simulink model "solution1"  (R2017b)
settings: Solver=VariableStepAuto  StartTime=0.0  StopTime=25  FixedStep=0.1  MaxStep=1e-1  RelTol=1e-3  AbsTol=1e-3
libraries: simulink x7
settings Model: Creator=ashwin.ramanujam  LastModifiedBy=otkup

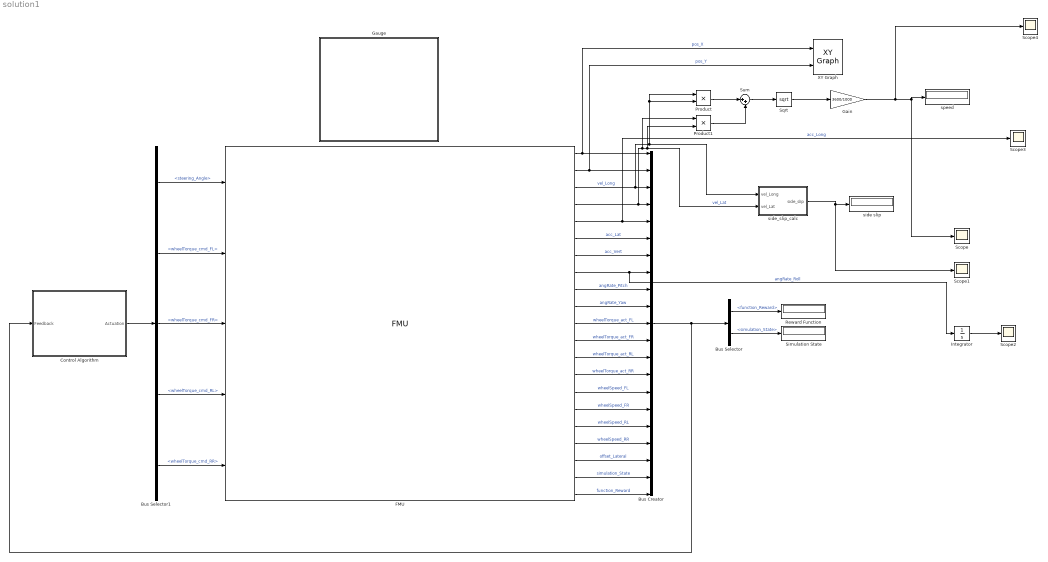
== system solution1 ==
  Bus Creator : BusCreator  Inputs=21
  Bus Selector : BusSelector  OutputSignals=function_Reward,simulation_State
  Bus Selector1 : BusSelector  OutputSignals=steering_Angle,wheelTorque_cmd_FL,wheelTorque_cmd_FR,wheelTorque_cmd_RL,wheelTorque_cmd_RR
  Control Algorithm : Subsystem
  FMU : FMU  FMUName=MED2018_VehicleModel.fmu  FMUDebugLogging=on  FMUMode=CoSimulation  FMUSampleTime=-1  mask(MED2018.VehicleModel [Co-Simulation, v2.0]){}
      mask Display:
      | if (exist([Simulink.fileGenControl('get','CacheFolder') '\slprj\_fmu\e4d23254ffb0d907ce810887e987e94d\MED2018_VehicleModel\model.png'],'file'))
      |     image([Simulink.fileGenControl('get','CacheFolder') '\slprj\_fmu\e4d23254ffb0d907ce810887e987e94d\MED2018_VehicleModel\model.png']);
      |     text(0.03, 0.97, 'MED2018.VehicleModel', 'horizontalAlignment', 'left', 'verticalAlignment', 'top');
      | else
      |     disp('MED2018.VehicleModel');
      | end
      | port_label('output',1,'pos_X');
      | port_label('output',2,'pos_Y');
      | port_label('output',3,'vel_Long');
      | port_label('output',4,'vel_Lat');
      | port_label('output',5,'acc_Long');
      | port_label('output',6,'acc_Lat');
      | port_label('output',7,'acc_Vert');
      | port_label('output',8,'angRate_Roll');
      | port_label('output',9,'angRate_Pitch');
      | port_label('output',10,'angRate_Yaw');
      | port_label('output',11,'wheellTorque_act_FL');
      | port_label('output',12,'wheelTorque_act_FR');
      | port_label('output',13,'wheelTorque_act_RL');
      | port_label('output',14,'wheelTorque_act_RR');
      | port_label('output',15,'wheelSpeed_FL');
      | port_label('output',16,'wheelSpeed_FR');
      | port_label('output',17,'wheelSpeed_RL');
      | port_label('output',18,'wheelSpeed_RR');
      | port_label('output',19,'offset_Lateral');
      | port_label('output',20,'simulation_State');
      | port_label('output',21,'function_Reward');
      | port_label('input',1,'steering_Angle');
      | port_label('input',2,'wheelTorque_cmd_FL');
      | port_label('input',3,'wheelTorque_cmd_FR');
      | port_label('input',4,'wheelTorque_cmd_RL');
      | port_label('input',5,'wheelTorque_cmd_RR');
  Gain : Gain  Gain=3600/1000
  Gauge : Subsystem  DialogController=hmiCreateDDGDialog  IsWebBlock=on  mask(MWDashboardBlock){webBlockId=95ecb222-2df1-432b-9766-14efc8d26a24, webBlockType=circulargauge, ShowInLibBrowser=on, ShowInitialText=on, HMISrcModelName=solution1}
      mask prompts: webBlockId "WebBlock Id"; webBlockType "WebBlock Type"; HMISrcModelName "Source Model"
      mask help: SimulinkHMI:dialogs:CircularGaugeDialogDesc
      mask Help: helpview([docroot '/mapfiles/simulink.map'], 'hmi_gauge')
      mask Display:
      | if strcmp(get_param(bdroot(gcb),'BlockDiagramType'), 'library')
      |     image([(matlabroot) '/toolbox/simulink/hmi/icons/CircularGauge.png']);
      | end
  Integrator : Integrator
  Product : Product
  Product1 : Product
  Reward Function : Display
  Scope{,1..4} (5 alike) : Scope
  Simulation State : Display
  Sqrt : Sqrt  SaturateOnIntegerOverflow=on
  Sum : Sum  Inputs=|++
  XY Graph : simulink/Sinks/XY Graph  xmin=-100  xmax=200  ymin=-100  ymax=200  st=-1
  "side slip " : Display
  side_slip_calc : Subsystem
  "speed " : Display
  wires:
  Control Algorithm/1(Actuation) -> Bus Selector1/1
  Bus Selector1/1 -> FMU/1  "<steering_Angle>"
  Bus Selector1/2 -> FMU/2  "<wheelTorque_cmd_FL>"
  Bus Selector1/3 -> FMU/3  "<wheelTorque_cmd_FR>"
  Bus Selector1/4 -> FMU/4  "<wheelTorque_cmd_RL>"
  Bus Selector1/5 -> FMU/5  "<wheelTorque_cmd_RR>"
  FMU/1 -> XY Graph/1, Bus Creator/1  "pos_X"
  FMU/2 -> XY Graph/2, Bus Creator/2  "pos_Y"
  FMU/3 -> side_slip_calc/1(vel_Long), Product/2, Product/1, Bus Creator/3  "vel_Long"
  FMU/4 -> Product1/1, side_slip_calc/2(vel_Lat), Product1/2, Bus Creator/4  "vel_Lat"
  FMU/5 -> Scope3/1, Bus Creator/5  "acc_Long"
  FMU/6 -> Bus Creator/6  "acc_Lat"
  FMU/7 -> Bus Creator/7  "acc_Vert"
  FMU/8 -> Integrator/1, Bus Creator/8  "angRate_Roll"
  FMU/9 -> Bus Creator/9  "angRate_Pitch"
  FMU/10 -> Bus Creator/10  "angRate_Yaw"
  FMU/11 -> Bus Creator/11  "wheelTorque_act_FL"
  FMU/12 -> Bus Creator/12  "wheelTorque_act_FR"
  FMU/13 -> Bus Creator/13  "wheelTorque_act_RL"
  FMU/14 -> Bus Creator/14  "wheelTorque_act_RR"
  FMU/15 -> Bus Creator/15  "wheelSpeed_FL"
  FMU/16 -> Bus Creator/16  "wheelSpeed_FR"
  FMU/17 -> Bus Creator/17  "wheelSpeed_RL"
  FMU/18 -> Bus Creator/18  "wheelSpeed_RR"
  FMU/19 -> Bus Creator/19  "offset_Lateral"
  FMU/20 -> Bus Creator/20  "simulation_State"
  FMU/21 -> Bus Creator/21  "function_Reward"
  Bus Creator/1 -> Bus Selector/1, Control Algorithm/1(Feedback)
  Bus Selector/1 -> Reward Function/1  "<function_Reward>"
  Bus Selector/2 -> Simulation State/1  "<simulation_State>"
  Product1/1 -> Sum/2
  Product/1 -> Sum/1
  Sum/1 -> Sqrt/1
  Sqrt/1 -> Gain/1
  Gain/1 -> Scope4/1, "speed "/1, Scope/1
  Integrator/1 -> Scope2/1
  side_slip_calc/1(side_slip) -> Scope1/1, "side slip "/1

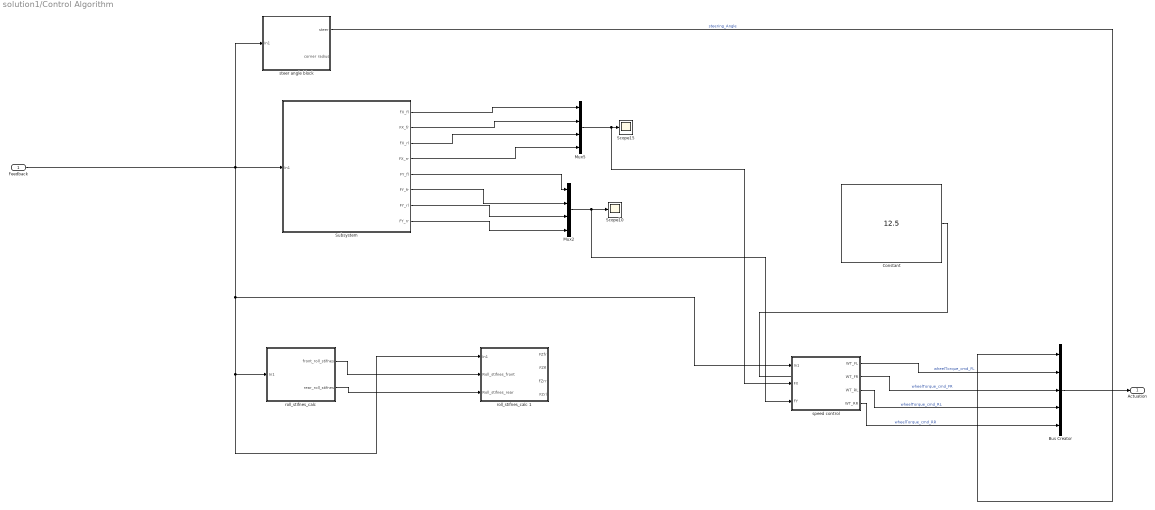
== system solution1/Control Algorithm ==
  Feedback : Inport
  Bus Creator : BusCreator  Inputs=5
  Constant : Constant  Value=12.5
  Mux2 : Mux
  Mux5 : Mux
  Scope10 : Scope
  Scope15 : Scope
  Subsystem : Subsystem
  "roll_stifnes_calc " : Subsystem
  roll_stifnes_calc 1 : Subsystem
  speed control : Subsystem
  "steer angle block " : Subsystem
  Actuation : Outport
  wires:
  speed control/4(WT_RR) -> Bus Creator/5  "wheelTorque_cmd_RR"
  speed control/1("WT_FL ") -> Bus Creator/2  "wheelTorque_cmd_FL"
  speed control/3(WT_RL) -> Bus Creator/4  "wheelTorque_cmd_RL"
  "steer angle block "/1("steer ") -> Bus Creator/1  "steering_Angle"
  speed control/2(WT_FR) -> Bus Creator/3  "wheelTorque_cmd_FR"
  Bus Creator/1 -> Actuation/1
  "roll_stifnes_calc "/1(front_roll_stifnes) -> roll_stifnes_calc 1/2(Roll_stifnes_front)
  "roll_stifnes_calc "/2(rear_roll_stifnes) -> roll_stifnes_calc 1/3("Roll_stifnes_rear ")
  Feedback/1 -> speed control/1(In1), roll_stifnes_calc 1/1(In1), "roll_stifnes_calc "/1(In1), "steer angle block "/1(In1), Subsystem/1(In1)
  Constant/1 -> ?
  Mux5/1 -> speed control/2(FX), Scope15/1
  Mux2/1 -> speed control/3(FY), Scope10/1
  Subsystem/1(FX_fl) -> Mux5/1
  Subsystem/2(FX_fr) -> Mux5/2
  Subsystem/3(FX_rl) -> Mux5/3
  Subsystem/4(FX_rr) -> Mux5/4
  Subsystem/5(FY_fl) -> Mux2/1
  Subsystem/6(FY_fr) -> Mux2/2
  Subsystem/7(FY_rl) -> Mux2/3
  Subsystem/8(FY_rr) -> Mux2/4

== system solution1/Gauge ==

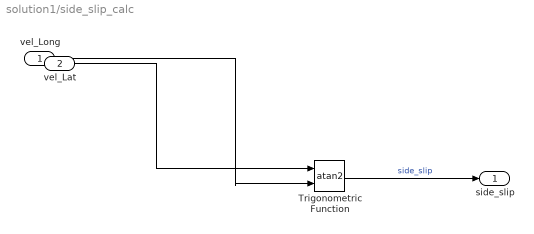
== system solution1/side_slip_calc ==
  vel_Long : Inport
  vel_Lat : Inport  Port=2
  Trigonometric Function : Trigonometry  Operator=atan2
  side_slip : Outport
  wires:
  Trigonometric Function/1 -> side_slip/1  "side_slip"
  vel_Lat/1 -> Trigonometric Function/1
  vel_Long/1 -> Trigonometric Function/2

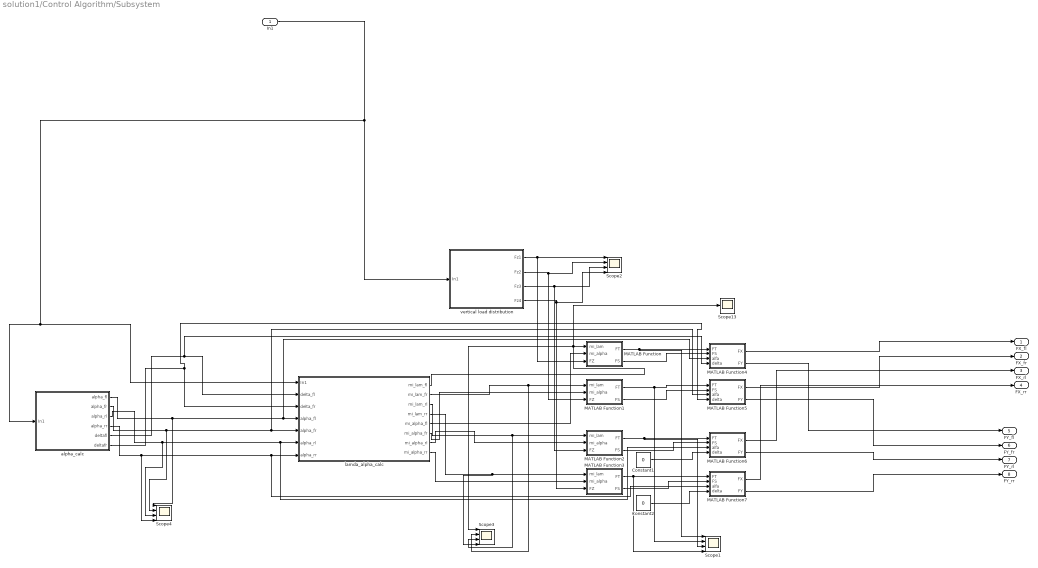
== system solution1/Control Algorithm/Subsystem ==
  In1 : Inport
  Constant1 : Constant  Value=0
  Constant2 : Constant  Value=0
  MATLAB Function : MATLAB Function  TreatAsAtomicUnit=on
  MATLAB Function1 : MATLAB Function  TreatAsAtomicUnit=on
  MATLAB Function2 : MATLAB Function  TreatAsAtomicUnit=on
  MATLAB Function3 : MATLAB Function  TreatAsAtomicUnit=on
  MATLAB Function4 : MATLAB Function  TreatAsAtomicUnit=on
  MATLAB Function5 : MATLAB Function  TreatAsAtomicUnit=on
  MATLAB Function6 : MATLAB Function  TreatAsAtomicUnit=on
  MATLAB Function7 : MATLAB Function  TreatAsAtomicUnit=on
  Scope{1..4} (4 alike) : Scope  NumInputPorts=4
  Scope13 : Scope
  alpha_calc : Subsystem
  lamda_alpha_calc : Subsystem
  vertical load distribution : Subsystem
  FX_fl : Outport
  FX_fr : Outport  Port=2
  FX_rl : Outport  Port=3
  FX_rr : Outport  Port=4
  FY_fl : Outport  Port=5
  FY_fr : Outport  Port=6
  FY_rl : Outport  Port=7
  FY_rr : Outport  Port=8
  wires:
  MATLAB Function/1(FT) -> Scope1/1, MATLAB Function4/1(FT)
  MATLAB Function6/2(FY) -> FY_rl/1
  MATLAB Function4/1(FX) -> FX_fl/1
  MATLAB Function6/1(FX) -> FX_rl/1
  MATLAB Function4/2(FY) -> FY_fl/1
  Constant1/1 -> MATLAB Function6/4(delta)
  vertical load distribution/3(Fz3) -> Scope2/3, MATLAB Function2/3(FZ)
  vertical load distribution/2(Fz2) -> Scope2/2, MATLAB Function1/3(FZ)
  alpha_calc/5(deltafl) -> MATLAB Function4/4(delta), lamda_alpha_calc/2(delta_fl)
  alpha_calc/6(deltafr) -> MATLAB Function5/4(delta), lamda_alpha_calc/3(delta_fr)
  vertical load distribution/4(Fz4) -> Scope2/4, MATLAB Function3/3(FZ)
  vertical load distribution/1(Fz1) -> Scope2/1, MATLAB Function/3(FZ)
  alpha_calc/3(alpha_rl) -> Scope4/3, MATLAB Function6/3(alfa), lamda_alpha_calc/6(alpha_rl)
  alpha_calc/2(alpha_fr) -> Scope4/2, MATLAB Function5/3(alfa), lamda_alpha_calc/5(alpha_fr)
  alpha_calc/4(alpha_rr) -> Scope4/4, MATLAB Function7/3(alfa), lamda_alpha_calc/7(alpha_rr)
  MATLAB Function3/1(FT) -> Scope1/4, MATLAB Function7/1(FT)
  MATLAB Function2/2(FS) -> MATLAB Function6/2(FS)
  MATLAB Function1/2(FS) -> MATLAB Function5/2(FS)
  MATLAB Function/2(FS) -> MATLAB Function4/2(FS)
  lamda_alpha_calc/4(mi_lam_rr) -> Scope3/4, MATLAB Function3/1(mi_lam)
  MATLAB Function5/1(FX) -> FX_fr/1
  MATLAB Function7/1(FX) -> FX_rr/1
  MATLAB Function5/2(FY) -> FY_fr/1
  lamda_alpha_calc/2(mi_lam_fr) -> Scope3/2, MATLAB Function1/1(mi_lam)
  lamda_alpha_calc/6(mi_alpha_fr) -> MATLAB Function1/2(mi_alpha)
  MATLAB Function7/2(FY) -> FY_rr/1
  MATLAB Function2/1(FT) -> Scope1/3, MATLAB Function6/1(FT)
  MATLAB Function1/1(FT) -> Scope1/2, MATLAB Function5/1(FT)
  lamda_alpha_calc/5(mi_alpha_fl) -> MATLAB Function/2(mi_alpha)
  In1/1 -> alpha_calc/1(In1), lamda_alpha_calc/1(In1), vertical load distribution/1(In1)
  lamda_alpha_calc/7(mi_alpha_rl) -> MATLAB Function2/2(mi_alpha)
  lamda_alpha_calc/3(mi_lam_rl) -> Scope3/3, MATLAB Function2/1(mi_lam)
  lamda_alpha_calc/8(mi_alpha_rr) -> MATLAB Function3/2(mi_alpha)
  MATLAB Function3/2(FS) -> MATLAB Function7/2(FS)
  Constant2/1 -> MATLAB Function7/4(delta)
  lamda_alpha_calc/1("mi_lam_fl ") -> Scope3/1, Scope13/1, MATLAB Function/1(mi_lam)
  alpha_calc/1(alpha_fl) -> Scope4/1, MATLAB Function4/3(alfa), lamda_alpha_calc/4(alpha_fl)

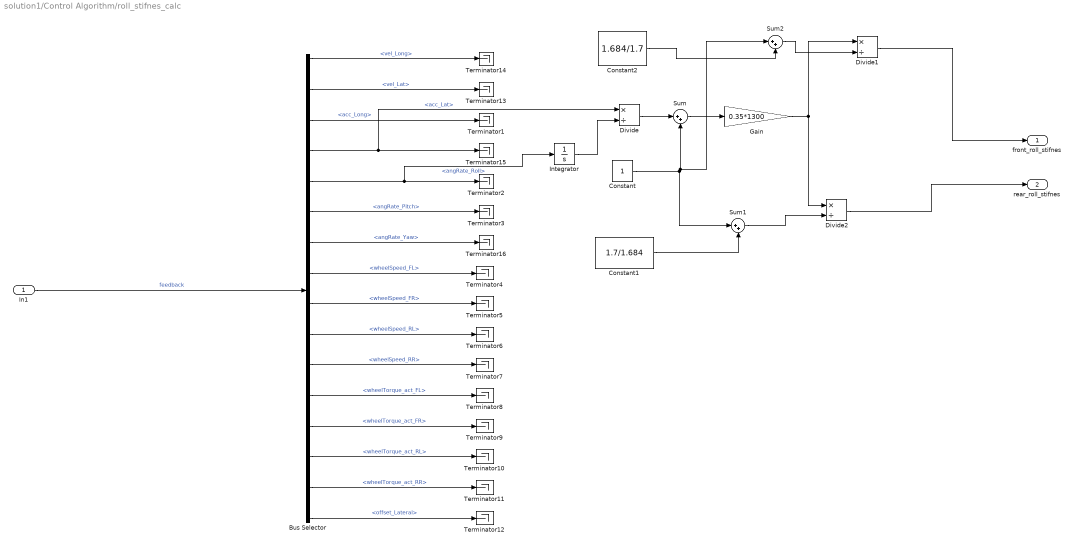
== system solution1/Control Algorithm/roll_stifnes_calc  ==
  In1 : Inport
  Bus Selector : BusSelector  OutputSignals=vel_Long,vel_Lat,acc_Long,acc_Lat,angRate_Roll,angRate_Pitch,angRate_Yaw,wheelSpeed_FL,wheelSpeed_FR,wheelSpeed_RL,wheelSpeed_RR,wheelTorque_act_FL,wheelTorque_act_FR,wheelTorque_act_RL,wheelTorque_act_RR,offset_Lateral
  Constant : Constant
  Constant1 : Constant  Value=1.7/1.684
  Constant2 : Constant  Value=1.684/1.7
  Divide : Product  Inputs=*/
  Divide1 : Product  Inputs=*/
  Divide2 : Product  Inputs=*/
  Gain : Gain  Gain=0.35*1300
  Integrator : Integrator
  Sum : Sum  Inputs=|++
  Sum1 : Sum  Inputs=|++
  Sum2 : Sum  Inputs=|++
  Terminator{1..16} (16 alike) : Terminator
  front_roll_stifnes : Outport
  rear_roll_stifnes : Outport  Port=2
  wires:
  Bus Selector/7 -> Terminator16/1  "<angRate_Yaw>"
  Bus Selector/4 -> Divide/1, Terminator15/1  "<acc_Lat>"
  Bus Selector/1 -> Terminator14/1  "<vel_Long>"
  In1/1 -> Bus Selector/1  "feedback"
  Bus Selector/13 -> Terminator9/1  "<wheelTorque_act_FR>"
  Bus Selector/5 -> Integrator/1, Terminator2/1  "<angRate_Roll>"
  Bus Selector/14 -> Terminator10/1  "<wheelTorque_act_RL>"
  Bus Selector/11 -> Terminator7/1  "<wheelSpeed_RR>"
  Bus Selector/12 -> Terminator8/1  "<wheelTorque_act_FL>"
  Bus Selector/16 -> Terminator12/1  "<offset_Lateral>"
  Bus Selector/15 -> Terminator11/1  "<wheelTorque_act_RR>"
  Bus Selector/9 -> Terminator5/1  "<wheelSpeed_FR>"
  Bus Selector/8 -> Terminator4/1  "<wheelSpeed_FL>"
  Bus Selector/10 -> Terminator6/1  "<wheelSpeed_RL>"
  Bus Selector/6 -> Terminator3/1  "<angRate_Pitch>"
  Bus Selector/3 -> Terminator1/1  "<acc_Long>"
  Bus Selector/2 -> Terminator13/1  "<vel_Lat>"
  Integrator/1 -> Divide/2
  Constant/1 -> Sum1/1, Sum2/1, Sum/2
  Divide/1 -> Sum/1
  Sum/1 -> Gain/1
  Gain/1 -> Divide2/1, Divide1/1
  Sum2/1 -> Divide1/2
  Sum1/1 -> Divide2/2
  Constant1/1 -> Sum1/2
  Constant2/1 -> Sum2/2
  Divide1/1 -> front_roll_stifnes/1
  Divide2/1 -> rear_roll_stifnes/1

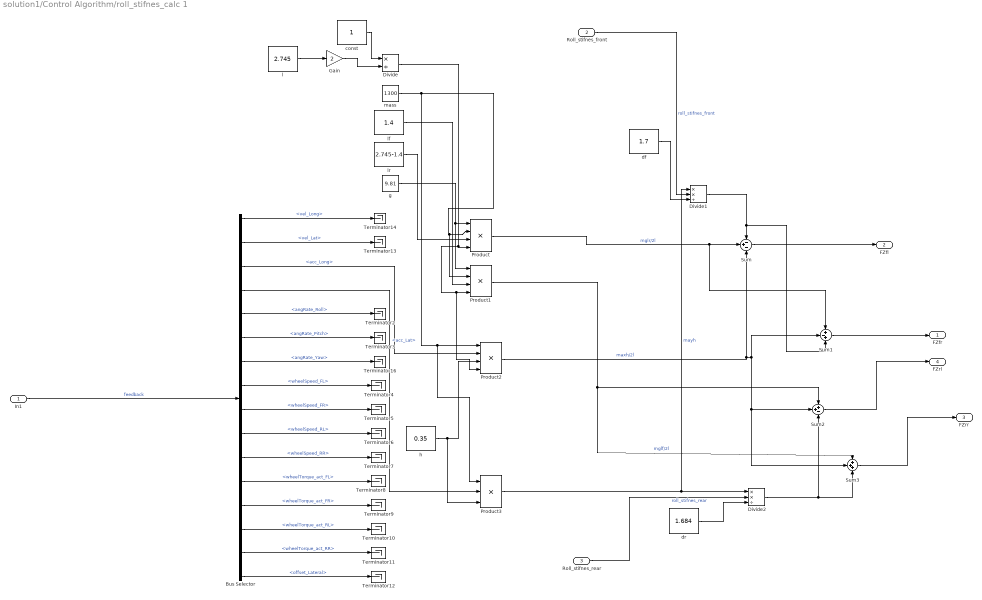
== system solution1/Control Algorithm/roll_stifnes_calc 1 ==
  In1 : Inport
  Roll_stifnes_front : Inport  Port=2
  "Roll_stifnes_rear " : Inport  Port=3
  Bus Selector : BusSelector  OutputSignals=vel_Long,vel_Lat,acc_Long,acc_Lat,angRate_Roll,angRate_Pitch,angRate_Yaw,wheelSpeed_FL,wheelSpeed_FR,wheelSpeed_RL,wheelSpeed_RR,wheelTorque_act_FL,wheelTorque_act_FR,wheelTorque_act_RL,wheelTorque_act_RR,offset_Lateral
  Divide : Product  Inputs=*/
  Divide1 : Product  Inputs=**/
  Divide2 : Product  Inputs=**/
  Gain : Gain  Gain=2
  Product : Product  Inputs=4
  Product1 : Product  Inputs=4
  Product2 : Product  Inputs=4
  Product3 : Product  Inputs=3
  Sum : Sum  Inputs=-+-
  Sum1 : Sum  Inputs=+-+
  Sum2 : Sum  Inputs=++-
  Sum3 : Sum  Inputs=+++
  Terminator{2..14,16} (14 alike) : Terminator
  const : Constant
  df : Constant  Value=1.7
  dr : Constant  Value=1.684
  g : Constant  Value=9.81
  h : Constant  Value=0.35
  "l " : Constant  Value=2.745
  "lf " : Constant  Value=1.4
  lr : Constant  Value=2.745-1.4
  mass : Constant  Value=1300
  FZfr : Outport
  FZfl : Outport  Port=2
  FZrr : Outport  Port=3
  FZrl : Outport  Port=4
  wires:
  Bus Selector/2 -> Terminator13/1  "<vel_Lat>"
  Bus Selector/3 -> Product2/2  "<acc_Long>"
  Bus Selector/6 -> Terminator3/1  "<angRate_Pitch>"
  Bus Selector/10 -> Terminator6/1  "<wheelSpeed_RL>"
  Bus Selector/8 -> Terminator4/1  "<wheelSpeed_FL>"
  Bus Selector/9 -> Terminator5/1  "<wheelSpeed_FR>"
  Bus Selector/15 -> Terminator11/1  "<wheelTorque_act_RR>"
  Bus Selector/16 -> Terminator12/1  "<offset_Lateral>"
  Bus Selector/12 -> Terminator8/1  "<wheelTorque_act_FL>"
  Bus Selector/11 -> Terminator7/1  "<wheelSpeed_RR>"
  Bus Selector/14 -> Terminator10/1  "<wheelTorque_act_RL>"
  Bus Selector/5 -> Terminator2/1  "<angRate_Roll>"
  Bus Selector/13 -> Terminator9/1  "<wheelTorque_act_FR>"
  In1/1 -> Bus Selector/1  "feedback"
  Bus Selector/1 -> Terminator14/1  "<vel_Long>"
  Bus Selector/4 -> Product3/2  "<acc_Lat>"
  Bus Selector/7 -> Terminator16/1  "<angRate_Yaw>"
  Roll_stifnes_front/1 -> Divide1/2  "roll_stifnes_front"
  "Roll_stifnes_rear "/1 -> Divide2/2  "roll_stifnes_rear"
  g/1 -> Product1/1, Product/1
  mass/1 -> Product3/1, Product2/1, Product1/2, Product/2
  lr/1 -> Product/3
  "lf "/1 -> Product1/3
  Product1/1 -> Sum3/1, Sum2/1  "mglf/2l"
  "l "/1 -> Gain/1
  const/1 -> Divide/1
  Gain/1 -> Divide/2
  Divide/1 -> Product2/4, Product1/4, Product/4
  h/1 -> Product3/3, Product2/3
  Product2/1 -> Sum3/2, Sum2/2, Sum1/2, Sum/3  "maxh/2l"
  Product3/1 -> Divide2/1, Divide1/1  "mayh"
  Sum/1 -> FZfl/1
  Product/1 -> Sum1/1, Sum/2  "mglr/2l"
  df/1 -> Divide1/3
  Divide1/1 -> Sum1/3, Sum/1
  Sum1/1 -> FZfr/1
  Sum2/1 -> FZrl/1
  Divide2/1 -> Sum3/3, Sum2/3
  dr/1 -> Divide2/3
  Sum3/1 -> FZrr/1

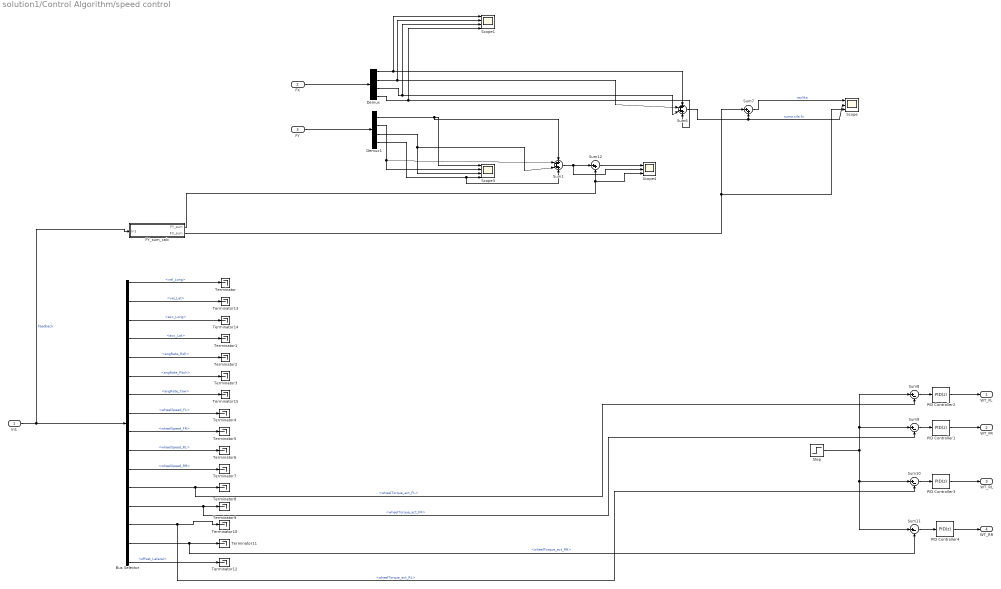
== system solution1/Control Algorithm/speed control ==
  In1 : Inport
  FX : Inport  Port=2
  FY : Inport  Port=3
  Bus Selector : BusSelector  OutputSignals=vel_Long,vel_Lat,acc_Long,acc_Lat,angRate_Roll,angRate_Pitch,angRate_Yaw,wheelSpeed_FL,wheelSpeed_FR,wheelSpeed_RL,wheelSpeed_RR,wheelTorque_act_FL,wheelTorque_act_FR,wheelTorque_act_RL,wheelTorque_act_RR,offset_Lateral
  Demux : Demux
  Demux1 : Demux
  FY_sum_calc : Subsystem
  PID Controller{1..4} (4 alike) : simulink/Continuous/PID Controller  Controller=PID  TimeDomain=Discrete-time  SampleTime=-1  IntegratorMethod=Forward Euler  FilterMethod=Forward Euler  Form=Parallel  UseFilter=on  ControllerParametersSource=internal  P=1  I=1.5  D=0  N=100  InitialConditionSource=internal  InitialConditionForIntegrator=0  InitialConditionForFilter=0  ExternalReset=none  LimitOutput=off  UpperSaturationLimit=inf  LowerSaturationLimit=-inf  LinearizeAsGain=on  AntiWindupMode=none  Kb=1  TrackingMode=off  Kt=1  PParamMin=[]  PParamMax=[]  IParamMin=[]  IParamMax=[]  DParamMin=[]  DParamMax=[]  NParamMin=[]  NParamMax=[]  KbParamMin=[]  KbParamMax=[]  KtParamMin=[]  KtParamMax=[]  POutMin=[]  POutMax=[]  IOutMin=[]  IOutMax=[]  DOutMin=[]  DOutMax=[]  NOutMin=[]  NOutMax=[]  KbOutMin=[]  KbOutMax=[]  KtOutMin=[]  KtOutMax=[]  IntegratorOutMin=[]  IntegratorOutMax=[]  FilterOutMin=[]  FilterOutMax=[]  SumOutMin=[]  SumOutMax=[]  SumI1OutMin=[]  SumI1OutMax=[]  SumI2OutMin=[]  SumI2OutMax=[]  SumI3OutMin=[]  SumI3OutMax=[]  SumDOutMin=[]  SumDOutMax=[]  SaturationOutMin=[]  SaturationOutMax=[]  IntegratorContinuousStateAttributes=''  IntegratorStateMustResolveToSignalObject=off  IntegratorRTWStateStorageClass=Auto  FilterContinuousStateAttributes=''  FilterStateMustResolveToSignalObject=off  FilterRTWStateStorageClass=Auto  DifferentiatorICPrevScaledInput=0  DifferentiatorOutMin=[]  DifferentiatorOutMax=[]  InitialConditionSetting=State (most efficient)  FilterDiffOutCoefMin=[]  FilterDiffOutCoefMax=[]  SumDenOutMin=[]  SumDenOutMax=[]  SumNumOutMin=[]  SumNumOutMax=[]  ReciprocalOutMin=[]  ReciprocalOutMax=[]  DivideOutMin=[]  DivideOutMax=[]  TunerSelectOption=Transfer Function Based (PID Tuner App)
  Scope : Scope  NumInputPorts=3
  Scope1 : Scope  NumInputPorts=4
  Scope3 : Scope  NumInputPorts=4
  Scope4 : Scope  NumInputPorts=3
  Step : Step  Time=15  Before=12.5  After=1000  SampleTime=0
  Sum1 : Sum  Inputs=++++
  Sum{8..11} (4 alike) : Sum  Inputs=|+-
  Sum12 : Sum  Inputs=|++
  Sum6 : Sum  Inputs=++++
  Sum7 : Sum  Inputs=|++
  Terminator{,1..15} (16 alike) : Terminator
  "WT_FL " : Outport
  WT_FR : Outport  Port=2
  WT_RL : Outport  Port=3
  WT_RR : Outport  Port=4
  wires:
  Bus Selector/7 -> Terminator15/1  "<angRate_Yaw>"
  Bus Selector/2 -> Terminator13/1  "<vel_Lat>"
  Bus Selector/3 -> Terminator14/1  "<acc_Long>"
  Bus Selector/6 -> Terminator3/1  "<angRate_Pitch>"
  Bus Selector/10 -> Terminator6/1  "<wheelSpeed_RL>"
  Bus Selector/8 -> Terminator4/1  "<wheelSpeed_FL>"
  Bus Selector/9 -> Terminator5/1  "<wheelSpeed_FR>"
  Bus Selector/15 -> Sum11/2, Terminator11/1  "<wheelTorque_act_RR>"
  Bus Selector/16 -> Terminator12/1  "<offset_Lateral>"
  Bus Selector/12 -> Sum8/2, Terminator8/1  "<wheelTorque_act_FL>"
  Bus Selector/11 -> Terminator7/1  "<wheelSpeed_RR>"
  Bus Selector/14 -> Sum10/2, Terminator10/1  "<wheelTorque_act_RL>"
  Bus Selector/1 -> Terminator/1  "<vel_Long>"
  Bus Selector/5 -> Terminator2/1  "<angRate_Roll>"
  Bus Selector/13 -> Sum9/2, Terminator9/1  "<wheelTorque_act_FR>"
  Bus Selector/4 -> Terminator1/1  "<acc_Lat>"
  In1/1 -> FY_sum_calc/1(In1), Bus Selector/1  "feedback"
  FX/1 -> Demux/1
  FY/1 -> Demux1/1
  Demux/1 -> Scope1/1, Sum6/1
  Demux/2 -> Scope1/2, Sum6/2
  Demux/3 -> Scope1/3, Sum6/3
  Sum7/1 -> Scope/1  "razlika"
  Sum6/1 -> Scope/2, Sum7/2  "suma sila fx"
  Sum10/1 -> PID Controller3/1
  Sum11/1 -> PID Controller4/1
  Sum9/1 -> PID Controller1/1
  Sum8/1 -> PID Controller2/1
  Step/1 -> Sum10/1, Sum11/1, Sum9/1, Sum8/1
  PID Controller2/1 -> "WT_FL "/1
  PID Controller1/1 -> WT_FR/1
  PID Controller3/1 -> WT_RL/1
  PID Controller4/1 -> WT_RR/1
  Demux/4 -> Scope1/4, Sum6/4
  Demux1/1 -> Sum1/1, Scope3/1
  Demux1/2 -> Sum1/2, Scope3/2
  Demux1/3 -> Sum1/3, Scope3/3
  Demux1/4 -> Sum1/4, Scope3/4
  Sum1/1 -> Scope4/2, Sum12/1
  FY_sum_calc/1(FY_sum) -> Scope4/3, Sum12/2
  Sum12/1 -> Scope4/1
  FY_sum_calc/2(FX_sum) -> Scope/3, Sum7/1

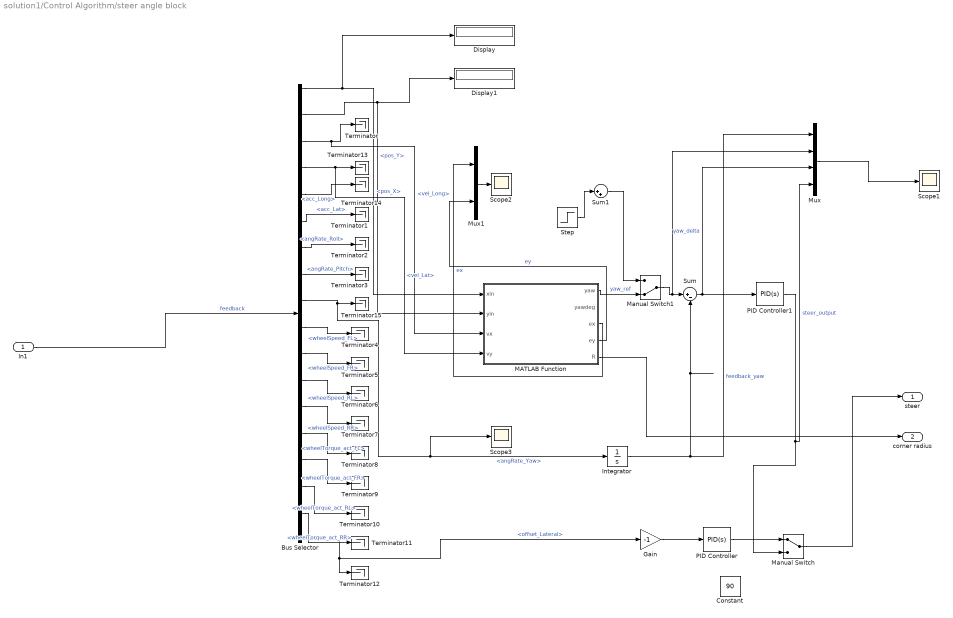
== system solution1/Control Algorithm/steer angle block  ==
  In1 : Inport
  Bus Selector : BusSelector  OutputSignals=pos_X,pos_Y,vel_Long,vel_Lat,acc_Long,acc_Lat,angRate_Roll,angRate_Pitch,angRate_Yaw,wheelSpeed_FL,wheelSpeed_FR,wheelSpeed_RL,wheelSpeed_RR,wheelTorque_act_FL,wheelTorque_act_FR,wheelTorque_act_RL,wheelTorque_act_RR,offset_Lateral
  Constant : Constant  Value=90
  Display : Display
  Display1 : Display
  Gain : Gain  Gain=-1
  Integrator : Integrator
  MATLAB Function : MATLAB Function  TreatAsAtomicUnit=on
  Manual Switch : ManualSwitch
  Manual Switch1 : ManualSwitch  CurrentSetting=0
  Mux : Mux
  Mux1 : Mux  Inputs=2
  PID Controller : simulink/Continuous/PID Controller  Controller=PID  TimeDomain=Continuous-time  SampleTime=-1  IntegratorMethod=Forward Euler  FilterMethod=Forward Euler  Form=Parallel  UseFilter=on  ControllerParametersSource=internal  P=1  I=0  D=1  N=100  InitialConditionSource=internal  InitialConditionForIntegrator=0  InitialConditionForFilter=0  ExternalReset=none  LimitOutput=off  UpperSaturationLimit=inf  LowerSaturationLimit=-inf  LinearizeAsGain=on  AntiWindupMode=none  Kb=1  TrackingMode=off  Kt=1  PParamMin=[]  PParamMax=[]  IParamMin=[]  IParamMax=[]  DParamMin=[]  DParamMax=[]  NParamMin=[]  NParamMax=[]  KbParamMin=[]  KbParamMax=[]  KtParamMin=[]  KtParamMax=[]  POutMin=[]  POutMax=[]  IOutMin=[]  IOutMax=[]  DOutMin=[]  DOutMax=[]  NOutMin=[]  NOutMax=[]  KbOutMin=[]  KbOutMax=[]  KtOutMin=[]  KtOutMax=[]  IntegratorOutMin=[]  IntegratorOutMax=[]  FilterOutMin=[]  FilterOutMax=[]  SumOutMin=[]  SumOutMax=[]  SumI1OutMin=[]  SumI1OutMax=[]  SumI2OutMin=[]  SumI2OutMax=[]  SumI3OutMin=[]  SumI3OutMax=[]  SumDOutMin=[]  SumDOutMax=[]  SaturationOutMin=[]  SaturationOutMax=[]  IntegratorContinuousStateAttributes=''  IntegratorStateMustResolveToSignalObject=off  IntegratorRTWStateStorageClass=Auto  FilterContinuousStateAttributes=''  FilterStateMustResolveToSignalObject=off  FilterRTWStateStorageClass=Auto  DifferentiatorICPrevScaledInput=0  DifferentiatorOutMin=[]  DifferentiatorOutMax=[]  InitialConditionSetting=State (most efficient)  FilterDiffOutCoefMin=[]  FilterDiffOutCoefMax=[]  SumDenOutMin=[]  SumDenOutMax=[]  SumNumOutMin=[]  SumNumOutMax=[]  ReciprocalOutMin=[]  ReciprocalOutMax=[]  DivideOutMin=[]  DivideOutMax=[]  TunerSelectOption=Transfer Function Based (PID Tuner App)
  PID Controller1 : simulink/Continuous/PID Controller  Controller=PID  TimeDomain=Continuous-time  SampleTime=-1  IntegratorMethod=Forward Euler  FilterMethod=Forward Euler  Form=Parallel  UseFilter=on  ControllerParametersSource=internal  P=12  I=0  D=0.2  N=0  InitialConditionSource=internal  InitialConditionForIntegrator=0  InitialConditionForFilter=0  ExternalReset=none  LimitOutput=off  UpperSaturationLimit=inf  LowerSaturationLimit=-inf  LinearizeAsGain=on  AntiWindupMode=none  Kb=1  TrackingMode=off  Kt=1  PParamMin=[]  PParamMax=[]  IParamMin=[]  IParamMax=[]  DParamMin=[]  DParamMax=[]  NParamMin=[]  NParamMax=[]  KbParamMin=[]  KbParamMax=[]  KtParamMin=[]  KtParamMax=[]  POutMin=[]  POutMax=[]  IOutMin=[]  IOutMax=[]  DOutMin=[]  DOutMax=[]  NOutMin=[]  NOutMax=[]  KbOutMin=[]  KbOutMax=[]  KtOutMin=[]  KtOutMax=[]  IntegratorOutMin=[]  IntegratorOutMax=[]  FilterOutMin=[]  FilterOutMax=[]  SumOutMin=[]  SumOutMax=[]  SumI1OutMin=[]  SumI1OutMax=[]  SumI2OutMin=[]  SumI2OutMax=[]  SumI3OutMin=[]  SumI3OutMax=[]  SumDOutMin=[]  SumDOutMax=[]  SaturationOutMin=[]  SaturationOutMax=[]  IntegratorContinuousStateAttributes=''  IntegratorStateMustResolveToSignalObject=off  IntegratorRTWStateStorageClass=Auto  FilterContinuousStateAttributes=''  FilterStateMustResolveToSignalObject=off  FilterRTWStateStorageClass=Auto  DifferentiatorICPrevScaledInput=0  DifferentiatorOutMin=[]  DifferentiatorOutMax=[]  InitialConditionSetting=State (most efficient)  FilterDiffOutCoefMin=[]  FilterDiffOutCoefMax=[]  SumDenOutMin=[]  SumDenOutMax=[]  SumNumOutMin=[]  SumNumOutMax=[]  ReciprocalOutMin=[]  ReciprocalOutMax=[]  DivideOutMin=[]  DivideOutMax=[]  TunerSelectOption=Transfer Function Based (PID Tuner App)
  Scope1 : Scope
  Scope2 : Scope
  Scope3 : Scope
  Step : Step  Time=0  After=0  SampleTime=0
  Sum : Sum  Inputs=|+-
  Sum1 : Sum  Inputs=|++
  Terminator{,1..15} (16 alike) : Terminator
  "steer " : Outport
  corner radius : Outport  Port=2
  wires:
  In1/1 -> Bus Selector/1  "feedback"
  Bus Selector/6 -> Terminator1/1  "<acc_Lat>"
  Bus Selector/15 -> Terminator9/1  "<wheelTorque_act_FR>"
  Bus Selector/7 -> Terminator2/1  "<angRate_Roll>"
  Bus Selector/3 -> MATLAB Function/3(vx), Terminator/1  "<vel_Long>"
  Bus Selector/16 -> Terminator10/1  "<wheelTorque_act_RL>"
  Bus Selector/13 -> Terminator7/1  "<wheelSpeed_RR>"
  Bus Selector/14 -> Terminator8/1  "<wheelTorque_act_FL>"
  Bus Selector/18 -> Terminator12/1, Gain/1  "<offset_Lateral>"
  Bus Selector/17 -> Terminator11/1  "<wheelTorque_act_RR>"
  Bus Selector/11 -> Terminator5/1  "<wheelSpeed_FR>"
  Bus Selector/10 -> Terminator4/1  "<wheelSpeed_FL>"
  Bus Selector/12 -> Terminator6/1  "<wheelSpeed_RL>"
  Bus Selector/8 -> Terminator3/1  "<angRate_Pitch>"
  Bus Selector/5 -> Terminator14/1  "<acc_Long>"
  Bus Selector/9 -> Scope3/1, Integrator/1, Terminator15/1  "<angRate_Yaw>"
  Gain/1 -> PID Controller/1
  PID Controller/1 -> Manual Switch/1
  Manual Switch/1 -> "steer "/1
  Integrator/1 -> Mux/1, Sum/2  "feedback_yaw"
  Sum/1 -> PID Controller1/1, Mux/3  "yaw_delta"
  Bus Selector/1 -> Display/1, MATLAB Function/1(xin)  "<pos_X>"
  Bus Selector/2 -> MATLAB Function/2(yin), Display1/1  "<pos_Y>"
  Bus Selector/4 -> MATLAB Function/4(vy), Terminator13/1  "<vel_Lat>"
  PID Controller1/1 -> Mux/4, Manual Switch/2  "steer_output"
  Mux/1 -> Scope1/1
  MATLAB Function/3(ex) -> Mux1/1  "ex"
  MATLAB Function/4(ey) -> Mux1/2  "ey"
  Mux1/1 -> Scope2/1
  MATLAB Function/1(yaw) -> Manual Switch1/2  "yaw_ref"
  Manual Switch1/1 -> Mux/2, Sum/1
  Step/1 -> Sum1/1
  Sum1/1 -> Manual Switch1/1
  MATLAB Function/5(R) -> corner radius/1

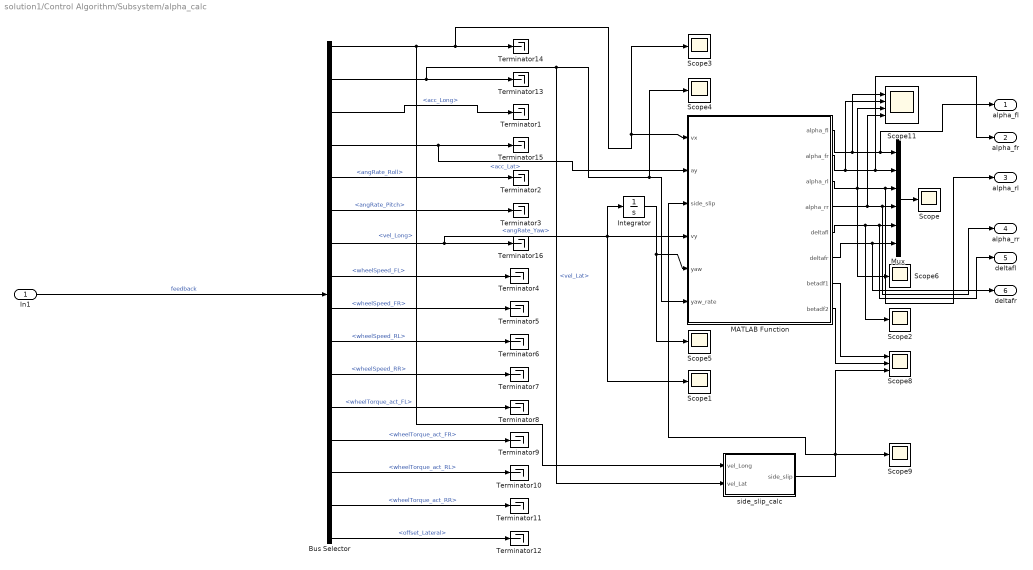
== system solution1/Control Algorithm/Subsystem/alpha_calc ==
  In1 : Inport
  Bus Selector : BusSelector  OutputSignals=vel_Long,vel_Lat,acc_Long,acc_Lat,angRate_Roll,angRate_Pitch,angRate_Yaw,wheelSpeed_FL,wheelSpeed_FR,wheelSpeed_RL,wheelSpeed_RR,wheelTorque_act_FL,wheelTorque_act_FR,wheelTorque_act_RL,wheelTorque_act_RR,offset_Lateral
  Integrator : Integrator
  MATLAB Function : MATLAB Function  TreatAsAtomicUnit=on
  Mux : Mux  Inputs=6
  Scope{,1..6,9} (8 alike) : Scope
  Scope11 : Scope  NumInputPorts=4
  Scope8 : Scope  NumInputPorts=3
  Terminator{1..16} (16 alike) : Terminator
  side_slip_calc : Subsystem
  alpha_fl : Outport
  alpha_fr : Outport  Port=2
  alpha_rl : Outport  Port=3
  alpha_rr : Outport  Port=4
  deltafl : Outport  Port=5
  deltafr : Outport  Port=6
  wires:
  Bus Selector/7 -> Scope1/1, Integrator/1, MATLAB Function/6(yaw_rate), Terminator16/1  "<angRate_Yaw>"
  Bus Selector/4 -> MATLAB Function/2(ay), Terminator15/1  "<acc_Lat>"
  Bus Selector/1 -> side_slip_calc/1(vel_Long), Scope3/1, MATLAB Function/1(vx), Terminator14/1  "<vel_Long>"
  In1/1 -> Bus Selector/1  "feedback"
  Bus Selector/13 -> Terminator9/1  "<wheelTorque_act_FR>"
  Bus Selector/5 -> Terminator2/1  "<angRate_Roll>"
  Bus Selector/14 -> Terminator10/1  "<wheelTorque_act_RL>"
  Bus Selector/11 -> Terminator7/1  "<wheelSpeed_RR>"
  Bus Selector/12 -> Terminator8/1  "<wheelTorque_act_FL>"
  Bus Selector/16 -> Terminator12/1  "<offset_Lateral>"
  Bus Selector/15 -> Terminator11/1  "<wheelTorque_act_RR>"
  Bus Selector/9 -> Terminator5/1  "<wheelSpeed_FR>"
  Bus Selector/8 -> Terminator4/1  "<wheelSpeed_FL>"
  Bus Selector/10 -> Terminator6/1  "<wheelSpeed_RL>"
  Bus Selector/6 -> Terminator3/1  "<angRate_Pitch>"
  Bus Selector/3 -> Terminator1/1  "<acc_Long>"
  Bus Selector/2 -> side_slip_calc/2(vel_Lat), Scope4/1, MATLAB Function/4(vy), Terminator13/1  "<vel_Lat>"
  Integrator/1 -> Scope5/1, MATLAB Function/5(yaw)
  MATLAB Function/1(alpha_fl) -> alpha_fl/1, Mux/1, Scope11/1
  MATLAB Function/2(alpha_fr) -> Scope11/2, alpha_fr/1, Mux/2
  MATLAB Function/3(alpha_rl) -> Scope11/3, alpha_rl/1, Mux/3, Scope6/1
  MATLAB Function/4(alpha_rr) -> alpha_rr/1, Mux/4, Scope11/4
  MATLAB Function/5(deltafl) -> Scope2/1, deltafl/1, Mux/5
  Mux/1 -> Scope/1
  side_slip_calc/1(side_slip) -> Scope8/3, Scope9/1, MATLAB Function/3(side_slip)
  MATLAB Function/7(betadf1) -> Scope8/1
  MATLAB Function/8(betadf2) -> Scope8/2
  MATLAB Function/6(deltafr) -> deltafr/1, Mux/6

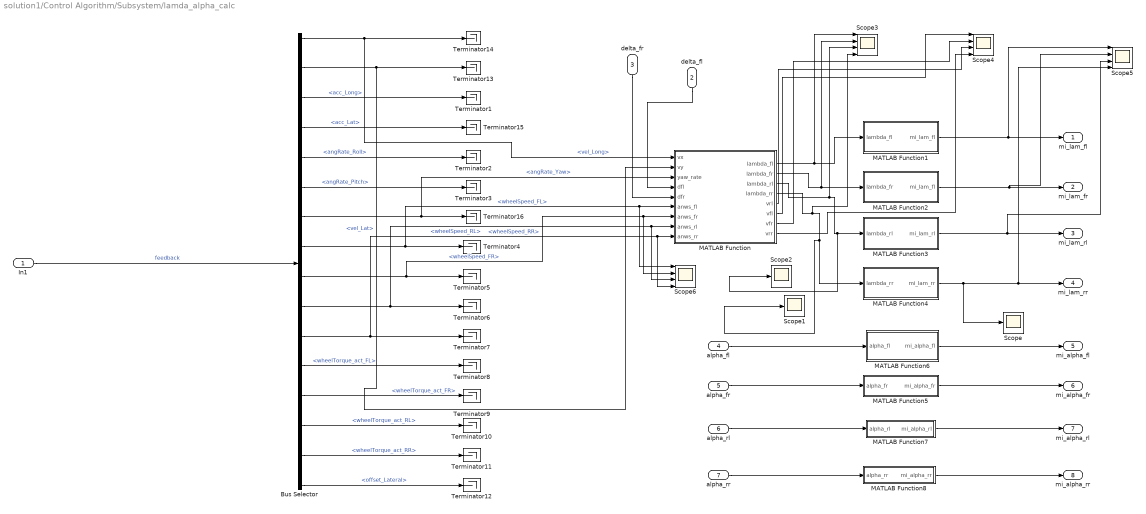
== system solution1/Control Algorithm/Subsystem/lamda_alpha_calc ==
  In1 : Inport
  delta_fl : Inport  Port=2
  delta_fr : Inport  Port=3
  alpha_fl : Inport  Port=4
  alpha_fr : Inport  Port=5
  alpha_rl : Inport  Port=6
  alpha_rr : Inport  Port=7
  Bus Selector : BusSelector  OutputSignals=vel_Long,vel_Lat,acc_Long,acc_Lat,angRate_Roll,angRate_Pitch,angRate_Yaw,wheelSpeed_FL,wheelSpeed_FR,wheelSpeed_RL,wheelSpeed_RR,wheelTorque_act_FL,wheelTorque_act_FR,wheelTorque_act_RL,wheelTorque_act_RR,offset_Lateral
  MATLAB Function : MATLAB Function  TreatAsAtomicUnit=on
  MATLAB Function1 : MATLAB Function  TreatAsAtomicUnit=on
  MATLAB Function2 : MATLAB Function  TreatAsAtomicUnit=on
  MATLAB Function3 : MATLAB Function  TreatAsAtomicUnit=on
  MATLAB Function4 : MATLAB Function  TreatAsAtomicUnit=on
  MATLAB Function5 : MATLAB Function  TreatAsAtomicUnit=on
  MATLAB Function6 : MATLAB Function  TreatAsAtomicUnit=on
  MATLAB Function7 : MATLAB Function  TreatAsAtomicUnit=on
  MATLAB Function8 : MATLAB Function  TreatAsAtomicUnit=on
  Scope : Scope
  Scope1 : Scope
  Scope2 : Scope
  Scope{3..6} (4 alike) : Scope  NumInputPorts=4
  Terminator{1..16} (16 alike) : Terminator
  "mi_lam_fl " : Outport
  mi_lam_fr : Outport  Port=2
  mi_lam_rl : Outport  Port=3
  mi_lam_rr : Outport  Port=4
  mi_alpha_fl : Outport  Port=5
  mi_alpha_fr : Outport  Port=6
  mi_alpha_rl : Outport  Port=7
  mi_alpha_rr : Outport  Port=8
  wires:
  Bus Selector/2 -> MATLAB Function/2(vy), Terminator13/1  "<vel_Lat>"
  Bus Selector/3 -> Terminator1/1  "<acc_Long>"
  Bus Selector/6 -> Terminator3/1  "<angRate_Pitch>"
  Bus Selector/10 -> Scope6/3, MATLAB Function/8(anws_rl), Terminator6/1  "<wheelSpeed_RL>"
  Bus Selector/8 -> Scope6/1, MATLAB Function/6(anws_fl), Terminator4/1  "<wheelSpeed_FL>"
  Bus Selector/9 -> Scope6/2, MATLAB Function/7(anws_fr), Terminator5/1  "<wheelSpeed_FR>"
  Bus Selector/15 -> Terminator11/1  "<wheelTorque_act_RR>"
  Bus Selector/16 -> Terminator12/1  "<offset_Lateral>"
  Bus Selector/12 -> Terminator8/1  "<wheelTorque_act_FL>"
  Bus Selector/11 -> Scope6/4, MATLAB Function/9(anws_rr), Terminator7/1  "<wheelSpeed_RR>"
  Bus Selector/14 -> Terminator10/1  "<wheelTorque_act_RL>"
  Bus Selector/5 -> Terminator2/1  "<angRate_Roll>"
  Bus Selector/13 -> Terminator9/1  "<wheelTorque_act_FR>"
  In1/1 -> Bus Selector/1  "feedback"
  Bus Selector/1 -> MATLAB Function/1(vx), Terminator14/1  "<vel_Long>"
  Bus Selector/4 -> Terminator15/1  "<acc_Lat>"
  Bus Selector/7 -> MATLAB Function/3(yaw_rate), Terminator16/1  "<angRate_Yaw>"
  delta_fl/1 -> MATLAB Function/4(dfl)
  delta_fr/1 -> MATLAB Function/5(dfr)
  MATLAB Function/1(lambda_fl) -> Scope3/1, MATLAB Function1/1(lambda_fl)
  MATLAB Function/2(lambda_fr) -> Scope3/2, MATLAB Function2/1(lambda_fr)
  MATLAB Function/4(lambda_rr) -> Scope3/4, Scope1/1, MATLAB Function4/1(lambda_rr)
  alpha_fl/1 -> MATLAB Function6/1(alpha_fl)
  alpha_fr/1 -> MATLAB Function5/1(alpha_fr)
  alpha_rl/1 -> MATLAB Function7/1(alpha_rl)
  alpha_rr/1 -> MATLAB Function8/1(alpha_rr)
  MATLAB Function1/1(mi_lam_fl) -> Scope5/1, "mi_lam_fl "/1
  MATLAB Function2/1(mi_lam_fl) -> Scope5/2, mi_lam_fr/1
  MATLAB Function3/1(mi_lam_rl) -> Scope5/3, mi_lam_rl/1
  MATLAB Function6/1(mi_alpha_fl) -> mi_alpha_fl/1
  MATLAB Function5/1(mi_alpha_fr) -> mi_alpha_fr/1
  MATLAB Function7/1(mi_alpha_rl) -> mi_alpha_rl/1
  MATLAB Function8/1(mi_alpha_rr) -> mi_alpha_rr/1
  MATLAB Function/3(lambda_rl) -> Scope3/3, Scope2/1, MATLAB Function3/1(lambda_rl)
  MATLAB Function/6(vfl) -> Scope4/1
  MATLAB Function/7(vfr) -> Scope4/2
  MATLAB Function/5(vrl) -> Scope4/3
  MATLAB Function/8(vrr) -> Scope4/4
  MATLAB Function4/1(mi_lam_rr) -> Scope/1, Scope5/4, mi_lam_rr/1

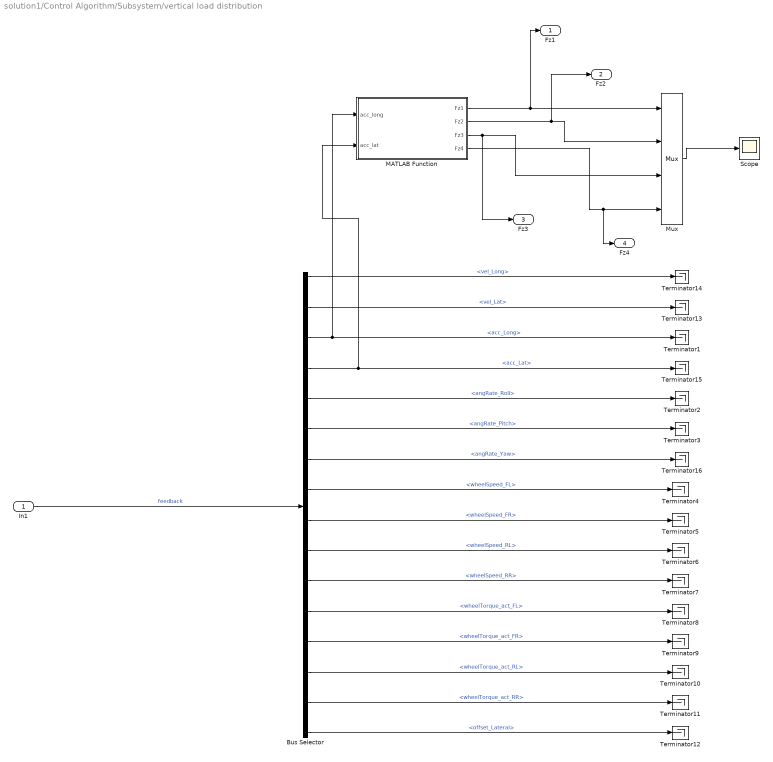
== system solution1/Control Algorithm/Subsystem/vertical load distribution ==
  In1 : Inport
  Bus Selector : BusSelector  OutputSignals=vel_Long,vel_Lat,acc_Long,acc_Lat,angRate_Roll,angRate_Pitch,angRate_Yaw,wheelSpeed_FL,wheelSpeed_FR,wheelSpeed_RL,wheelSpeed_RR,wheelTorque_act_FL,wheelTorque_act_FR,wheelTorque_act_RL,wheelTorque_act_RR,offset_Lateral
  MATLAB Function : MATLAB Function  TreatAsAtomicUnit=on
  Mux : Mux
  Scope : Scope
  Terminator{1..16} (16 alike) : Terminator
  Fz1 : Outport
  Fz2 : Outport  Port=2
  Fz3 : Outport  Port=3
  Fz4 : Outport  Port=4
  wires:
  Bus Selector/7 -> Terminator16/1  "<angRate_Yaw>"
  Bus Selector/1 -> Terminator14/1  "<vel_Long>"
  In1/1 -> Bus Selector/1  "feedback"
  Bus Selector/13 -> Terminator9/1  "<wheelTorque_act_FR>"
  Bus Selector/5 -> Terminator2/1  "<angRate_Roll>"
  Bus Selector/14 -> Terminator10/1  "<wheelTorque_act_RL>"
  Bus Selector/11 -> Terminator7/1  "<wheelSpeed_RR>"
  Bus Selector/12 -> Terminator8/1  "<wheelTorque_act_FL>"
  Bus Selector/16 -> Terminator12/1  "<offset_Lateral>"
  Bus Selector/15 -> Terminator11/1  "<wheelTorque_act_RR>"
  Bus Selector/9 -> Terminator5/1  "<wheelSpeed_FR>"
  Bus Selector/8 -> Terminator4/1  "<wheelSpeed_FL>"
  Bus Selector/10 -> Terminator6/1  "<wheelSpeed_RL>"
  Bus Selector/6 -> Terminator3/1  "<angRate_Pitch>"
  Bus Selector/3 -> MATLAB Function/1(acc_long), Terminator1/1  "<acc_Long>"
  Bus Selector/2 -> Terminator13/1  "<vel_Lat>"
  Mux/1 -> Scope/1
  MATLAB Function/1(Fz1) -> Fz1/1, Mux/1
  MATLAB Function/2(Fz2) -> Fz2/1, Mux/2
  MATLAB Function/3(Fz3) -> Fz3/1, Mux/3
  MATLAB Function/4(Fz4) -> Fz4/1, Mux/4
  Bus Selector/4 -> MATLAB Function/2(acc_lat), Terminator15/1  "<acc_Lat>"

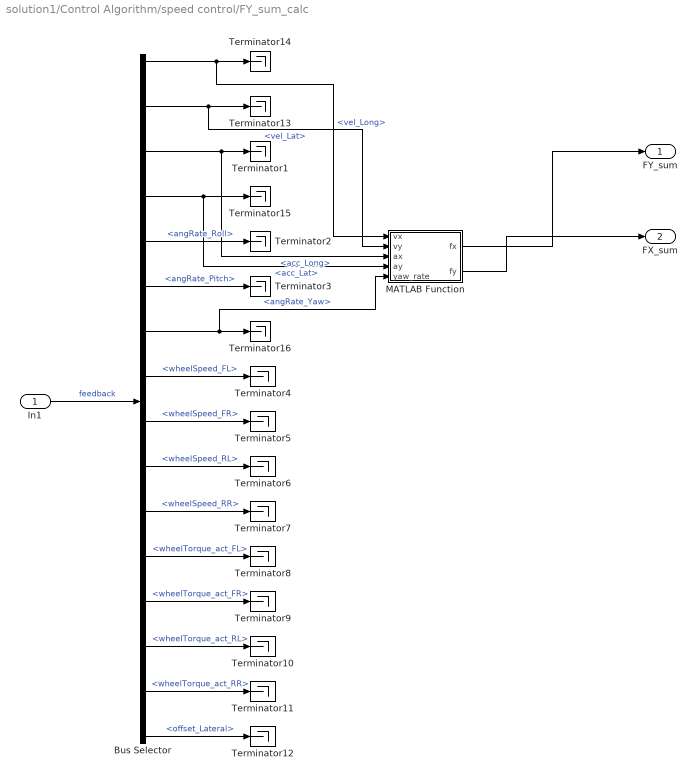
== system solution1/Control Algorithm/speed control/FY_sum_calc ==
  In1 : Inport
  Bus Selector : BusSelector  OutputSignals=vel_Long,vel_Lat,acc_Long,acc_Lat,angRate_Roll,angRate_Pitch,angRate_Yaw,wheelSpeed_FL,wheelSpeed_FR,wheelSpeed_RL,wheelSpeed_RR,wheelTorque_act_FL,wheelTorque_act_FR,wheelTorque_act_RL,wheelTorque_act_RR,offset_Lateral
  MATLAB Function : MATLAB Function  TreatAsAtomicUnit=on
  Terminator{1..16} (16 alike) : Terminator
  FY_sum : Outport
  FX_sum : Outport  Port=2
  wires:
  In1/1 -> Bus Selector/1  "feedback"
  Bus Selector/13 -> Terminator9/1  "<wheelTorque_act_FR>"
  Bus Selector/5 -> Terminator2/1  "<angRate_Roll>"
  Bus Selector/14 -> Terminator10/1  "<wheelTorque_act_RL>"
  Bus Selector/11 -> Terminator7/1  "<wheelSpeed_RR>"
  Bus Selector/12 -> Terminator8/1  "<wheelTorque_act_FL>"
  Bus Selector/16 -> Terminator12/1  "<offset_Lateral>"
  Bus Selector/15 -> Terminator11/1  "<wheelTorque_act_RR>"
  Bus Selector/9 -> Terminator5/1  "<wheelSpeed_FR>"
  Bus Selector/8 -> Terminator4/1  "<wheelSpeed_FL>"
  Bus Selector/10 -> Terminator6/1  "<wheelSpeed_RL>"
  Bus Selector/6 -> Terminator3/1  "<angRate_Pitch>"
  Bus Selector/3 -> MATLAB Function/3(ax), Terminator1/1  "<acc_Long>"
  Bus Selector/2 -> MATLAB Function/2(vy), Terminator13/1  "<vel_Lat>"
  Bus Selector/1 -> MATLAB Function/1(vx), Terminator14/1  "<vel_Long>"
  Bus Selector/4 -> MATLAB Function/4(ay), Terminator15/1  "<acc_Lat>"
  Bus Selector/7 -> MATLAB Function/5(yaw_rate), Terminator16/1  "<angRate_Yaw>"
  MATLAB Function/1(fx) -> FY_sum/1
  MATLAB Function/2(fy) -> FX_sum/1

== system solution1/Control Algorithm/Subsystem/alpha_calc/side_slip_calc ==
  vel_Long : Inport
  vel_Lat : Inport  Port=2
  Trigonometric Function : Trigonometry  Operator=atan2
  side_slip : Outport
  wires:
  Trigonometric Function/1 -> side_slip/1  "side_slip"
  vel_Lat/1 -> Trigonometric Function/1
  vel_Long/1 -> Trigonometric Function/2

== matlab function solution1/Control Algorithm/Subsystem/lamda_alpha_calc/MATLAB Function ==
  data: vx input; lambda_fl output; vy input; yaw_rate input; dfl input; dfr input; lambda_fr output; lambda_rl output; lambda_rr output; anws_fl input; anws_fr input; anws_rl input; anws_rr input; vrl output; vfl output; vfr output; vrr output
function [lambda_fl,lambda_fr,lambda_rl,lambda_rr,vrl,vfl,vfr,vrr] = lam_calc(vx,vy,yaw_rate,dfl,dfr,anws_fl,anws_fr,anws_rl,anws_rr)

lf=1.4
lr=2.745-1.4
tf=1.7
tr=1.684
rw=0.254

vfl=(vx-(tf/2)*yaw_rate)*cos(dfl)+(vy+lf*yaw_rate)*sin(dfl)
vfr=(vx+(tf/2)*yaw_rate)*cos(dfr)+(vy+lf*yaw_rate)*sin(dfr)

vrl=vx-(tr/2)*yaw_rate
vrr=vx+(tr/2)*yaw_rate

lambda_fl=(-rw*anws_fl+vfl)/(max([rw*anws_fl vfl]))
lambda_fr=(-rw*anws_fr+vfr)/(max([rw*anws_fr vfr]))

lambda_rl=(-rw*anws_rl+vrl)/(max([rw*anws_rl vrl]))
lambda_rr=(-rw*anws_rr+vrr)/(max([rw*anws_rr vrr]))



end

== matlab function solution1/Control Algorithm/steer angle block /MATLAB Function ==
  data: xin input; yin input; yaw output; vx input; yawdeg output; ex output; ey output; vy input; R output
function [yaw,yawdeg,ex,ey,R]  = yaw_calc(xin,yin, vx,vy)
%syms y  x x0 x1 y0 y1 r

%syms x y r
speed=sqrt(vx^2+vy^2)
step=speed/10
%% curve functions
%c1=50+sqrt(r^2-(y-50)^2)-x ;
%c2=50-sqrt(r^2-(y-135)^2)-x;


  ex=0
  ey=0
%% first part of track
if ((yin>-6)&(yin<6))&((xin>=0)&(xin<=50)) %%zalet
    disp('zalet')
    yaw=0;
    R=10000

elseif ((yin>-6)&(yin<120))&((xin>50)&(xin<200)) %%prvi zavoj
    R=50
    %p1=((yin-50)/(xin-50))*(x-50)+50-y
    %c11=subs(c1,r,50)
    disp('prvi zavoj')
    
    %[xc,yc]=solve([p1;c11])
    xc=[50-50*(1/(xin^2-100*xin+yin^2-100*yin+5000))^(1/2)*(xin-50) ; 50*(1/(xin^2-100*xin+yin^2-100*yin+5000))^(1/2)*(xin-50)+50] 
    yc=[50-50*(1/(xin^2-100*xin+yin^2-100*yin+5000))^(1/2)*(yin-50) ; 50*(1/(xin^2-100*xin+yin^2-100*yin+5000))^(1/2)*(yin-50)+50]
    ynew=yc(2)+step
    ynew=[ynew ynew]
    
    %xnew=subs(c1+x,[y r],[ynew 50])
    %xnew=subs(c1+x,[y r],[ynew 50])
    %disp('mark2')
    %xnew=[(2500-(ynew(1)-50)^2)^(1/2)+50 ; (2500-(ynew(2)-50)^2)^(1/2)+50]
    if(ynew(2)>100)
        ynew(2)=100
    end
    xnew=(2500-(ynew(2)-50)^2)^(1/2)+50
    xnew=[xnew xnew]
    %vpa([xc yc])
    %vpa([xnew ynew])
    
    %rjjjjj=(solve(c1,y))
    %disp('mark1')
    %cldiff=diff(solve(c1,y))
    cldiff1=[-(2*xnew(1)-100)/(2*(-xnew(1)*(xnew(1)-100))^(1/2)) ; (2*xnew(1)-100)/(2*(-xnew(1)*(xnew(1)-100))^(1/2))]
    %cldiff2=[-(2*xnew(2)-100)/(2*(-xnew(2)*(xnew(2)-100))^(1/2)) ; (2*xnew(2)-100)/(2*(-xnew(2)*(xnew(2)-100))^(1/2))]
    cldiff=[cldiff1(2)]%; cldiff2]
    if (not(xnew(1)==50+50))
    %tanyaw=subs(cldiff(2),[r x],[50 xnew])
    tanyaw=cldiff
    else
        tanyaw=inf
    end
    yaw=atand(tanyaw)
    if((xnew(2)<=100)&(ynew(2)>50))
        yaw=180-yaw
    end
    %vpa(yaw)
    %yaw=11;

    %ex=0
    %ey=0
    
elseif ((yin>94)&(yin<176))&((xin<=50)&(xin>9)) %%drugi zavoj
    R=-35
   %p2=((yin-135)/(xin-50))*(x-50)+135-y
   %c22=subs(c2,r,35)
    disp('drugi zavoj')
    %[xc,yc]=solve([p2;c22])
    xc=[50-35*(1/(xin^2-100*xin+yin^2-270*yin+20725))^(1/2)*(xin-50) ;   35*(1/(xin^2-100*xin+yin^2-270*yin+20725))^(1/2)*(xin-50)+50]
    yc=[135-35*(1/(xin^2-100*xin+yin^2-270*yin+20725))^(1/2)*(yin-135) ; 35*(1/(xin^2-100*xin+yin^2-270*yin+20725))^(1/2)*(yin-135)+135]
    ynew=yc+step
    ynew=[ynew(2) ynew(2)]
    disp('mark1')
    if ((ynew(1)>170)|(ynew(2)>170))
        ynew(1)=170
        ynew(2)=170
    end
    %xnew=subs(c2+x,[y r],[ynew 35])
    xnew=[50-(1225-(ynew(1)-135)^2)^(1/2) ; 50-(1225-(ynew(2)-135)^2)^(1/2)]
   
    %vpa([xc yc])
    %vpa([xnew ynew])
    disp('mark2')
    %cldiff=diff(solve(c2,y))
    cldiff1=[-(2*xnew(1)-100)/(2*(-(xnew(1)-15)*(xnew(1)-85))^(1/2)) ; (2*xnew(1)-100)/(2*(-(xnew(1)-15)*(xnew(1)-85))^(1/2))]
    cldiff2=[-(2*xnew(2)-100)/(2*(-(xnew(2)-15)*(xnew(2)-85))^(1/2)) ; (2*xnew(2)-100)/(2*(-(xnew(2)-15)*(xnew(2)-85))^(1/2))]
    
    cldiff=[cldiff1(1)]
    disp('mark3')
    if (not(xnew==50-35))
    tanyaw=cldiff
    else
        tanyaw=inf
    end
    yaw=atand(tanyaw)
    if((xnew(2)>15)&(ynew(2)>135))
        yaw=yaw
        disp('sl 2')
    else
        yaw=180-yaw
        disp('sl 1')
    end
    
    %kut=vpa(yaw)
    disp('drugi')
    %yaw=-11
    
    %ex=0
    %ey=0
elseif ((yin>94)&(yin<176))&((xin>50)&(xin<=100)) %zaustavljanje
    R=10000
    yaw=0
    ex=xin
    ey=yin
else
    R=10000
    yaw=55
    ex=xin
    ey=yin

end
yawdeg=yaw
yaw=yaw*pi/180


end

== matlab function solution1/Control Algorithm/Subsystem/lamda_alpha_calc/MATLAB Function1 ==
  data: lambda_fl input; mi_lam_fl output
function mi_lam_fl = friction_long_calc(lambda_fl)

xmax=0.1660
ymax=1.0612



mi_lam_fl = (2*ymax*xmax*lambda_fl)/(ymax^2+lambda_fl^2)

end

== matlab function solution1/Control Algorithm/Subsystem/alpha_calc/MATLAB Function ==
  data: vx input; ay input; side_slip input; alpha_fl output; vy input; yaw input; yaw_rate input; alpha_fr output; alpha_rl output; alpha_rr output; deltafl output; deltafr output; betadf1 output; betadf2 output
function [alpha_fl,alpha_fr,alpha_rl,alpha_rr,deltafl,deltafr,betadf1,betadf2] = lateral_slip_per_wheel(vx,ay,side_slip,vy,yaw,yaw_rate)
lf=1.4
lr=2.745-1.4
tf=1.7
tr=1.684

v=sqrt(vx^2+vy^2)

r=(v^2/ay)

alpha_rl=(atan((-lr*yaw_rate+vy)/(vx-tr/2*yaw_rate)))
alpha_rr=(atan((-lr*yaw_rate+vy)/(vx+tr/2*yaw_rate)))
alpha_fl=(atan((lf+lr)/(r-tf/2))-alpha_rl-((1/v)*9.81*vy))
%alpha_fl=55
alpha_fr=(atan((lf+lr)/(r+tf/2))-alpha_rr-((1/v)*9.81*vy))

deltafl=(atan((vy+yaw_rate*lr)/(vx-tf/2*yaw_rate))+alpha_fl)
deltafr=(atan((vy+yaw_rate*lr)/(vx+tf/2*yaw_rate))+alpha_fr)


alpha1=(atan((vy+yaw_rate*lr)/(vx-tf/2*yaw_rate))-deltafl)
alpha2=(atan((vy+yaw_rate*lr)/(vx+tf/2*yaw_rate))-deltafr)

alpha_fl=-alpha1
alpha_fr=-alpha2

betadf1=(deltafl-(lf*yaw_rate)/v+alpha1)
betadf2=(deltafr-(lf*yaw_rate)/v+alpha2)


end

== matlab function solution1/Control Algorithm/Subsystem/lamda_alpha_calc/MATLAB Function2 ==
  data: lambda_fr input; mi_lam_fl output
function mi_lam_fl = friction_long_calc(lambda_fr)

xmax=0.1660
ymax=1.0612



mi_lam_fl = (2*ymax*xmax*lambda_fr)/(ymax^2+lambda_fr^2)

end

== matlab function solution1/Control Algorithm/Subsystem/lamda_alpha_calc/MATLAB Function3 ==
  data: lambda_rl input; mi_lam_rl output
function mi_lam_rl = friction_long_calc(lambda_rl)

xmax=0.1660
ymax=1.0612



mi_lam_rl = (2*ymax*xmax*lambda_rl)/(ymax^2+lambda_rl^2)

end

== matlab function solution1/Control Algorithm/Subsystem/lamda_alpha_calc/MATLAB Function4 ==
  data: lambda_rr input; mi_lam_rr output
function mi_lam_rr = friction_long_calc(lambda_rr)

xmax=0.1660
ymax=1.0612



mi_lam_rr = (2*ymax*xmax*lambda_rr)/(ymax^2+lambda_rr^2)

end

== matlab function solution1/Control Algorithm/Subsystem/lamda_alpha_calc/MATLAB Function5 ==
  data: alpha_fr input; mi_alpha_fr output
function mi_alpha_fr = fcn(alpha_fr)
maxx=14.2170
maxy=0.9701

mi_alpha_fr=((2*maxx*maxy)/(maxx^2+alpha_fr^2))*alpha_fr


end

== matlab function solution1/Control Algorithm/Subsystem/lamda_alpha_calc/MATLAB Function6 ==
  data: alpha_fl input; mi_alpha_fl output
function mi_alpha_fl = fcn(alpha_fl)
maxx=14.2170
maxy=0.9701

mi_alpha_fl=((2*maxx*maxy)/(maxx^2+alpha_fl^2))*alpha_fl


end

== matlab function solution1/Control Algorithm/Subsystem/lamda_alpha_calc/MATLAB Function7 ==
  data: alpha_rl input; mi_alpha_rl output
function mi_alpha_rl = fcn(alpha_rl)
maxx=14.2170
maxy=0.9701

mi_alpha_rl=((2*maxx*maxy)/(maxx^2+alpha_rl^2))*alpha_rl


end

== matlab function solution1/Control Algorithm/Subsystem/lamda_alpha_calc/MATLAB Function8 ==
  data: alpha_rr input; mi_alpha_rr output
function mi_alpha_rr = fcn(alpha_rr)
maxx=14.2170
maxy=0.9701

mi_alpha_rr=((2*maxx*maxy)/(maxx^2+alpha_rr^2))*alpha_rr


end

== matlab function solution1/Control Algorithm/Subsystem/MATLAB Function ==
  data: mi_lam input; FT output; mi_alpha input; FZ input; FS output
function [FT,FS] = fcn(mi_lam,mi_alpha,FZ)
FT=FZ*mi_lam
FS=FZ*mi_alpha

end

== matlab function solution1/Control Algorithm/Subsystem/MATLAB Function1 ==
  data: mi_lam input; FT output; mi_alpha input; FZ input; FS output
function [FT,FS] = fcn(mi_lam,mi_alpha,FZ)
FT=FZ*mi_lam
FS=FZ*mi_alpha

end

== matlab function solution1/Control Algorithm/Subsystem/MATLAB Function2 ==
  data: mi_lam input; FT output; mi_alpha input; FZ input; FS output
function [FT,FS] = fcn(mi_lam,mi_alpha,FZ)
FT=FZ*mi_lam
FS=FZ*mi_alpha

end

== matlab function solution1/Control Algorithm/Subsystem/MATLAB Function3 ==
  data: mi_lam input; FT output; mi_alpha input; FZ input; FS output
function [FT,FS] = fcn(mi_lam,mi_alpha,FZ)
FT=FZ*mi_lam
FS=FZ*mi_alpha

end

== matlab function solution1/Control Algorithm/Subsystem/vertical load distribution/MATLAB Function ==
  data: acc_long input; Fz1 output; acc_lat input; Fz2 output; Fz3 output; Fz4 output
function [Fz1,Fz2,Fz3,Fz4] = fcn(acc_long,acc_lat)

l=2.745
mass=1300
lf=1.4
lr=2.745-1.4
g=9.81
h=0.35
tf=1.7
tr=1.684

Fz1=(lr*mass*g*cos(0))/(2*l)-(mass*acc_long)/(2*l)-(lr*h*mass*acc_lat)/(l*tr)
Fz2=(lr*mass*g*cos(0))/(2*l)-(mass*acc_long)/(2*l)+(lr*h*mass*acc_lat)/(l*tr)

Fz3=(lf*mass*g*cos(0))/(2*l)+(mass*acc_long)/(2*l)-(lf*h*mass*acc_lat)/(l*tf)
Fz4=(lf*mass*g*cos(0))/(2*l)+(mass*acc_long)/(2*l)+(lf*h*mass*acc_lat)/(l*tf)

end

== matlab function solution1/Control Algorithm/Subsystem/MATLAB Function4 ==
  data: FT input; FX output; FS input; alfa input; delta input; FY output
function [FX,FY] = fcn(FT,FS, alfa,delta)

FX=FT*cos(delta)-FS*sin(delta)*sign(alfa)
FY=FT*cos(delta)+FS*sin(delta)*sign(alfa)


end

== matlab function solution1/Control Algorithm/Subsystem/MATLAB Function5 ==
  data: FT input; FX output; FS input; alfa input; delta input; FY output
function [FX,FY] = fcn(FT,FS,alfa,delta)

FX=FT*cos(delta)-FS*sin(delta)*sign(alfa)
FY=FT*cos(delta)+FS*sin(delta)*sign(alfa)


end

== matlab function solution1/Control Algorithm/Subsystem/MATLAB Function6 ==
  data: FT input; FX output; FS input; alfa input; delta input; FY output
function [FX,FY] = fcn(FT,FS,alfa,delta)

FX=FT*cos(delta)-FS*sin(delta)*sign(alfa)
FY=FT*cos(delta)+FS*sin(delta)*sign(alfa)


end

== matlab function solution1/Control Algorithm/Subsystem/MATLAB Function7 ==
  data: FT input; FX output; FS input; alfa input; delta input; FY output
function [FX,FY] = fcn(FT,FS,alfa,delta)

FX=FT*cos(delta)-FS*sin(delta)*sign(alfa)
FY=FT*cos(delta)+FS*sin(delta)*sign(alfa)


end

== matlab function solution1/Control Algorithm/speed control/FY_sum_calc/MATLAB Function ==
  data: vx input; fx output; vy input; ax input; ay input; yaw_rate input; fy output
function [fx,fy] = fcn(vx,vy,ax,ay,yaw_rate)

m=1300

fx=m*(ax-yaw_rate*vy)
fy=m*(ay+yaw_rate*vx)

end
